simulink model "exp2_storageTank_ConstantFo"  (R2023a)
settings: Solver=VariableStepAuto  StartTime=0.0  StopTime=4  RelTol=1e-3
libraries: simulink x1
settings Model: Creator=Nipun_Work  LastModifiedBy=Nipun_Work

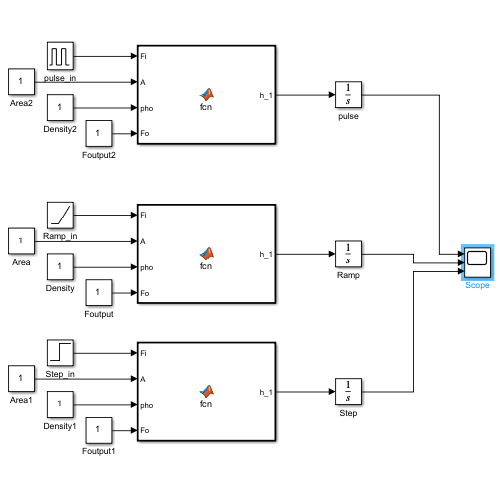
[thumbnail: Simulink's stored preview of the top-level diagram]
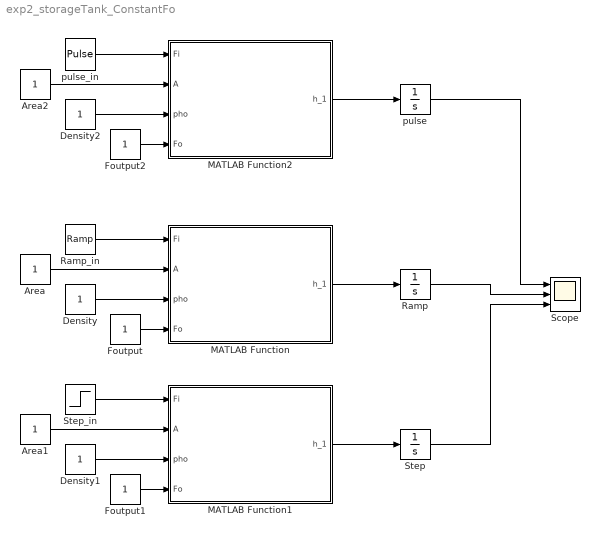
== system exp2_storageTank_ConstantFo ==
  Area : Constant
  Area1 : Constant
  Area2 : Constant
  Density : Constant
  Density1 : Constant
  Density2 : Constant
  Foutput : Constant
  Foutput1 : Constant
  Foutput2 : Constant
  MATLAB Function : MATLAB Function  TreatAsAtomicUnit=on
  MATLAB Function1 : MATLAB Function  TreatAsAtomicUnit=on
  MATLAB Function2 : MATLAB Function  TreatAsAtomicUnit=on
  Ramp : Integrator
  Ramp_in : simulink/Sources/Ramp  slope=0.5  start=0  InitialOutput=0
  Scope : Scope  NumInputPorts=3
  Step : Integrator
  Step_in : Step  SampleTime=0
  pulse : Integrator
  pulse_in : DiscretePulseGenerator  PulseType=Time based  Period=1  PulseWidth=60
  wires:
  Foutput/1 -> MATLAB Function/4(Fo)
  Density/1 -> MATLAB Function/3(pho)
  Area/1 -> MATLAB Function/2(A)
  MATLAB Function/1(h_1) -> Ramp/1
  Ramp/1 -> Scope/2
  Ramp_in/1 -> MATLAB Function/1(Fi)
  Density1/1 -> MATLAB Function1/3(pho)
  Area1/1 -> MATLAB Function1/2(A)
  Step_in/1 -> MATLAB Function1/1(Fi)
  Foutput1/1 -> MATLAB Function1/4(Fo)
  MATLAB Function1/1(h_1) -> Step/1
  MATLAB Function2/1(h_1) -> pulse/1
  Foutput2/1 -> MATLAB Function2/4(Fo)
  pulse_in/1 -> MATLAB Function2/1(Fi)
  Density2/1 -> MATLAB Function2/3(pho)
  Area2/1 -> MATLAB Function2/2(A)
  pulse/1 -> Scope/1
  Step/1 -> Scope/3

== matlab function exp2_storageTank_ConstantFo/MATLAB Function1 ==
  data: Fi input; h_1 output; A input; pho input; Fo input
function h_1 = fcn(Fi, A, pho, Fo)

h_1 = pho*(Fi-Fo)/(A*pho);

== matlab function exp2_storageTank_ConstantFo/MATLAB Function ==
  data: Fi input; h_1 output; A input; pho input; Fo input
function h_1 = fcn(Fi, A, pho, Fo)

h_1 = pho*(Fi-Fo)/(A*pho);

== matlab function exp2_storageTank_ConstantFo/MATLAB Function2 ==
  data: Fi input; h_1 output; A input; pho input; Fo input
function h_1 = fcn(Fi, A, pho, Fo)

h_1 = pho*(Fi-Fo)/(A*pho);
